simulink model "pendulo_mod_tarea"  (R2021a)
settings: Solver=ode45  StartTime=0.0  StopTime=60  MaxStep=1e-4  RelTol=1e-3  EnableMultiTasking=on
values from neighbouring files (symbols this model uses):
  b = 0.4    [Tp4.m]
  m = 1.1*mnom    (= 2.2)    [Tp4.m]
settings Model: Creator=Usuario  LastModifiedBy=bruno
settings SolverCC: AlgebraicLoopSolver=TrustRegion
settings DataIOCC: SaveFormat=Array  SignalLoggingSaveFormat=ModelDataLogs  ReturnWorkspaceOutputs=off
settings OptimizationCC: BlockReduction=off  BooleanDataType=off  InitFltsAndDblsToZero=on  LifeSpan=inf
settings DebuggingCC: SaveWithParameterizedLinksMsg=none  UnderspecifiedInitializationDetection=Classic  MergeDetectMultiDrivingBlocksExec=none  SignalResolutionControl=TryResolveAllWithWarning  MultiTaskDSMMsg=warning  MultiTaskCondExecSysMsg=none  FcnCallInpInsideContextMsg=warning  SFUnexpectedBacktrackingDiag=warning  SFNoUnconditionalDefaultTransitionDiag=warning  SFExecutionAtInitializationDiag=none  SFMachineParentedDataDiag=warning  ArithmeticOperatorsInVariantConditions=warning
settings HardwareCC: ProdBitPerPointer=32  ProdBitPerSizeT=32  ProdBitPerPtrDiffT=32  ProdLargestAtomicFloat=None  ProdIntDivRoundTo=Undefined  ProdEndianess=Unspecified  ProdWordSize=32  ProdHWDeviceType=32-bit Generic  TargetUnknown=on
settings ModelReferenceCC: PropagateSignalLabelsOutOfModel=off
settings SFSimCC: SimUseLocalCustomCode=off  CustomCodeUndefinedFunction=UseInterfaceOnly
settings RTWCC: RTWUseLocalCustomCode=off
settings CodeAppCC: StateflowObjectComments=on
settings GRTTargetCC: TargetFcnLib=ansi_tfl_tmw.mat  TargetLangStandard=C89/C90 (ANSI)  CombineOutputUpdateFcns=off  GRTInterface=on
settings ConfigComp: CovMetricSettings=dw  CovSaveCumulativeToWorkspaceVar=on  CovSaveSingleToWorkspaceVar=on  CovExternalEMLEnable=off  CovSFcnEnable=off

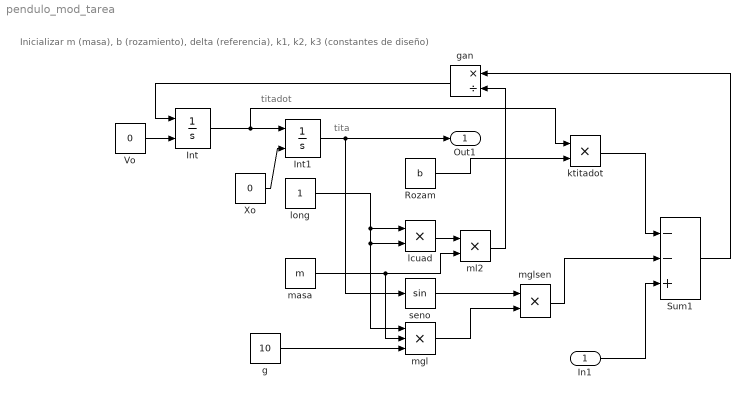
== system pendulo_mod_tarea ==
  note: Inicializar m (masa), b (rozamiento), delta (referencia), k1, k2, k3 (constantes de diseño)
  note: tita
  note: titadot
  In1 : Inport
  Int : Integrator  InitialConditionSource=external  InitialCondition=-10
  Int1 : Integrator  InitialConditionSource=external  InitialCondition=2.5
  Rozam : Constant  Value=b
  Sum1 : Sum  Inputs=--+  InputSameDT=on  SaturateOnIntegerOverflow=on  OutDataTypeStr=Inherit: Same as first input
  Vo : Constant  Value=0
  Xo : Constant  Value=0
  g : Constant  Value=10
  gan : Product  Inputs=*/
  ktitadot : Product  RndMeth=Zero
  lcuad : Product  RndMeth=Zero
  long : Constant
  masa : Constant  Value=m
  mgl : Product  Inputs=3  RndMeth=Zero
  mglsen : Product  RndMeth=Zero
  ml2 : Product  RndMeth=Zero
  seno : Trigonometry
  Out1 : Outport
  wires:
  Vo/1 -> Int/2
  Xo/1 -> Int1/2
  Int/1 -> Int1/1, ktitadot/1
  long/1 -> lcuad/1, lcuad/2, mgl/1
  masa/1 -> ml2/2, mgl/2
  lcuad/1 -> ml2/1
  Rozam/1 -> ktitadot/2
  ktitadot/1 -> Sum1/1
  g/1 -> mgl/3
  In1/1 -> Sum1/3
  mglsen/1 -> Sum1/2
  ml2/1 -> gan/2
  gan/1 -> Int/1
  mgl/1 -> mglsen/2
  seno/1 -> mglsen/1
  Sum1/1 -> gan/1
  Int1/1 -> Out1/1, seno/1
